simulink model "DCServoDAC"  (Simulink 8.9)
settings: Solver=ode4  StartTime=0.0  StopTime=5  RelTol=1e-3  EnableMultiTasking=on
undefined symbols (not defined in the file or in its folder): MIO, National_Instruments, PCI
libraries: sldrtlib x1
settings Model: Creator=Houska  LastModifiedBy=melab15  SimulationMode=external  ExtModeTrigDuration=10000
settings DataIOCC: SaveOutput=off  SignalLoggingName=logsOut
settings OptimizationCC: ExpressionDepthLimit=2147483647  InitFltsAndDblsToZero=on  LifeSpan=auto
settings DebuggingCC: SaveWithParameterizedLinksMsg=none  SignalResolutionControl=TryResolveAllWithWarning  MultiTaskDSMMsg=warning  MultiTaskCondExecSysMsg=none
settings HardwareCC: ProdBitPerPointer=64  ProdBitPerSizeT=64  ProdBitPerPtrDiffT=64  ProdLargestAtomicFloat=Float  ProdIntDivRoundTo=Zero  ProdEndianess=LittleEndian  ProdWordSize=64  ProdHWDeviceType=Intel->x86-64 (Windows64)
settings RTWCC: SystemTargetFile=sldrt.tlc  TemplateMakefile=sldrt.tmf  Description=Simulink Desktop Real-Time  RTWCompilerOptimization=on
settings CodeAppCC: MaxIdLength=95
settings SimulinkDesktopRealTimeCC: TargetFcnLib=ansi_tfl_tmw.mat  TargetPreCompLibLocation=C:\Program Files\MATLAB\R2017a\toolbox\sldrt\lib\win64  TargetLangStandard=C89/C90 (ANSI)  ModelReferenceCompliant=off  CompOptLevelCompliant=off  SupportVariableSizeSignals=off
settings ConfigComp: CovSFcnEnable=off

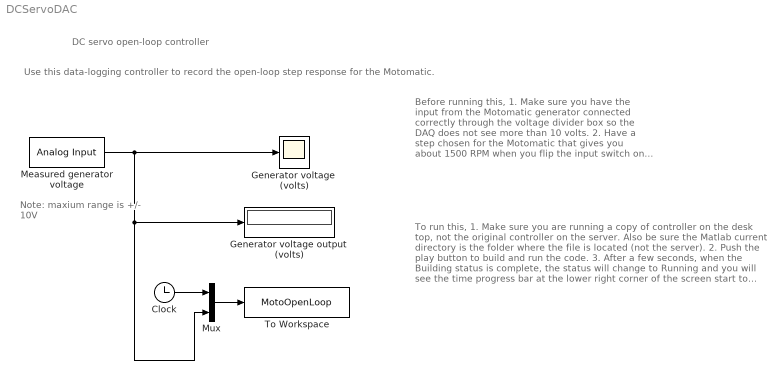
== system DCServoDAC ==
  note: Use this data-logging controller to record the open-loop step response for the Motomatic.
  note: Before running this,
      |
      | 1.  Make sure you have the input from the
      |     Motomatic generator connected correctly
      |     through the voltage divider box so the DAQ
      |     does not see more than 10 volts.
      | 2.  Have a step chosen for the Motomatic that
      |      gives you about 1500 RPM when you flip
      |     the input switch on (adjust this with the input
      |     knob on the Motomatic panel).
  note: To run this,
      |
      | 1.  Make sure you are running a copy of controller
      |     on the desk top, not the original controller on the
      |     server. Also be sure the Matlab current directory
      |      is the folder where the file is located (not the server).
      | 2.  Push the play button to build and run the code.
      | 3.  After a few seconds, when the Building status is complete,
      |      the status will change to Running and you will see the time progress
      |      bar at the lower right corner of the screen start to count
      |      off time. When it gets to about 1 second, then flip up the
      |      toggle switch on the Motomatic control box.
  note: DC servo open-loop controller
  note: Note: maxium range
      | is +/- 10V
  Clock : Clock
  Generator voltage output  (volts) : Display
  Generator voltage  (volts) : Scope
  Measured generator voltage : sldrtlib/Analog Input  SampleTime=1e-2  MaxMissedTicks=10  ShowMissedTicks=off  YieldWhenWaiting=off  DrvName=National_Instruments/PCI-MIO-16E-4  DrvAddress=4294967295  DrvOptions=[0 0 0 0 0]  Channels=2  RangeMode=1  VoltRange=1  DataType=1
      settings: AttributesFormatString=National Instruments\nPCI-MIO-16E-4 [auto]  SourceProductName=Simulink Desktop Real-Time
  Mux : Mux  Inputs=2
  To Workspace : ToWorkspace  VariableName=MotoOpenLoop  SampleTime=-1
  wires:
  Clock/1 -> Mux/1
  Measured generator voltage/1 -> Generator voltage  (volts)/1, Mux/2, Generator voltage output  (volts)/1
  Mux/1 -> To Workspace/1
